simulink model "RLC_S"  (R2020b)
settings: Solver=VariableStepAuto  StartTime=0.0  StopTime=30  FixedStep=1e-6  RelTol=1e-3
values from neighbouring files (symbols this model uses):
  c_r = 3.240869773689936e-07    (= 3.24086977369e-07)    [RLC_M.m]
  k_e = 0.023520507251362    (= 0.0235205072514)    [RLC_M.m]
  k_m = 0.022031575949394    (= 0.0220315759494)    [RLC_M.m]
  L = 1.754462619198655e-04    (= 0.00017544626192)    [RLC_M.m]    (also in as_labor03_const_u_motor_dc.m; as_labor04_hbridge.m)
  R = 3.263586106324851    (= 3.26358610632)    [RLC_M.m]    (also in as_labor01_2.m = 1/f2(1,1); as_labor03_const_u_motor_dc.m; as_labor04_hbridge.m)
  Uo = 8    [RLC_M.m]
settings Model: Creator=anton  LastModifiedBy=anton

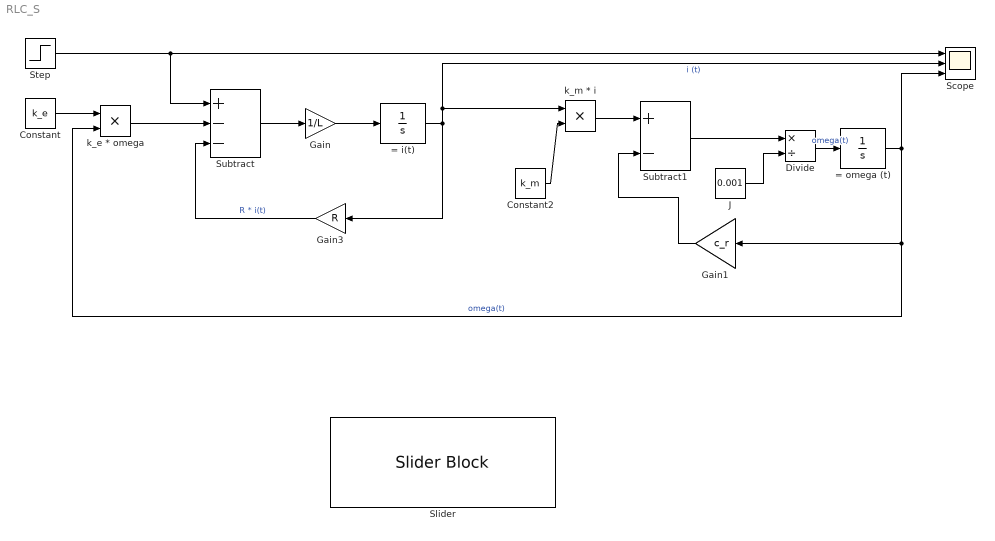
== system RLC_S ==
  " = i(t)" : Integrator
  = omega (t) : Integrator
  Constant : Constant  Value=k_e
  Constant2 : Constant  Value=k_m
  Divide : Product  Inputs=*/
  Gain : Gain  Gain=1/L
  Gain1 : Gain  Gain=c_r
  Gain3 : Gain  Gain=R
  J : Constant  Value=0.001
  Scope : Scope  NumInputPorts=3
  Slider : SliderBlock  ScaleMin=0e-4  ScaleMax=100e-4
  Step : Step  Time=0.1  After=Uo  SampleTime=0
  Subtract : Sum  Inputs=+--
  Subtract1 : Sum  Inputs=+-
  k_e * omega : Product
  k_m * i : Product
  wires:
  Constant/1 -> k_e * omega/1
  k_e * omega/1 -> Subtract/2
  Step/1 -> Scope/1, Subtract/1
  Gain3/1 -> Subtract/3  "R * i(t)"
  Subtract/1 -> Gain/1
  Gain/1 -> " = i(t)"/1
  " = i(t)"/1 -> Gain3/1, Scope/2, k_m * i/1  "i (t)"
  J/1 -> Divide/2
  Constant2/1 -> k_m * i/2
  k_m * i/1 -> Subtract1/1
  Gain1/1 -> Subtract1/2
  = omega (t)/1 -> Gain1/1, k_e * omega/2, Scope/3  "omega(t)"
  Subtract1/1 -> Divide/1
  Divide/1 -> = omega (t)/1  "omega(t)"
